simulink model "bug_nullpointer"  (Simulink 8.0)
settings: Solver=ode45  StartTime=0.0  StopTime=10.0  RelTol=1e-3
settings Model: Creator=ldnascim  LastModifiedBy=ldnascim

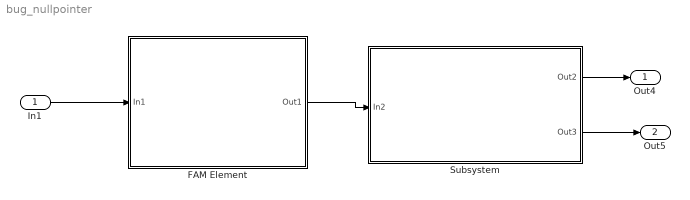
== system bug_nullpointer ==
  In1 : Inport
  FAM Element : Subsystem  Tag=FAM_Element
  Subsystem : Subsystem
  Out4 : Outport
  Out5 : Outport  Port=2
  wires:
  In1/1 -> FAM Element/1(In1)
  FAM Element/1(Out1) -> Subsystem/1(In2)
  Subsystem/1(Out2) -> Out4/1
  Subsystem/2(Out3) -> Out5/1

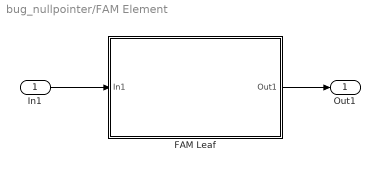
== system bug_nullpointer/FAM Element ==
  In1 : Inport
  FAM Leaf : Subsystem  Tag=FAM_Leaf  TreatAsAtomicUnit=on  mask{reqId=, dal=A, mdf=0, functionType=0}
      mask prompts: reqId "Requirement IDs"; dal "Design Assurance Level"; mdf "Minimum Design Frequency (Hz)"; functionType "Function type"
      mask init:
      | disp_text = compSys.fam.leaf.initialization(gcb);
      settings: MinAlgLoopOccurrences=on
      mask TypeOptions dal: A | B | C | D | E
      mask Callback functionType:
      | % This parameter is here to allow
      | % future compatibility with some
      | % specific function types, such as
      | % 'CAS Message' or 'Monitor'.
      | %
      | % Currently, it is not used.
      mask Display: disp(disp_text)
  Out1 : Outport
  wires:
  In1/1 -> FAM Leaf/1(In1)
  FAM Leaf/1(Out1) -> Out1/1

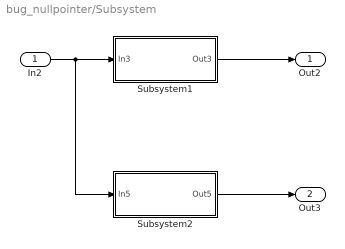
== system bug_nullpointer/Subsystem ==
  In2 : Inport
  Subsystem1 : Subsystem
  Subsystem2 : Subsystem
  Out2 : Outport
  Out3 : Outport  Port=2
  wires:
  In2/1 -> Subsystem2/1(In5), Subsystem1/1(In3)
  Subsystem1/1(Out3) -> Out2/1
  Subsystem2/1(Out5) -> Out3/1

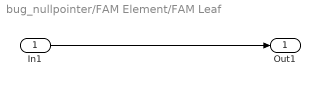
== system bug_nullpointer/FAM Element/FAM Leaf ==
  In1 : Inport
  Out1 : Outport
  wires:
  In1/1 -> Out1/1

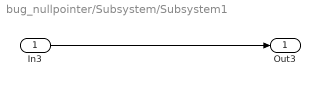
== system bug_nullpointer/Subsystem/Subsystem1 ==
  In3 : Inport
  Out3 : Outport
  wires:
  In3/1 -> Out3/1

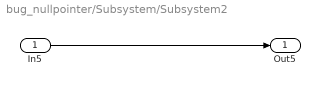
== system bug_nullpointer/Subsystem/Subsystem2 ==
  In5 : Inport
  Out5 : Outport
  wires:
  In5/1 -> Out5/1
